simulink model "myFirstRelayModel"  (R2022a)
settings: Solver=VariableStepAuto  StartTime=0.0  StopTime=H  RelTol=1e-3
values from neighbouring files (symbols this model uses):
  Ts = 1    [init.m]    (also in myFirstExtractedData.m; myFirstRelay.m = 0.1; myFirstRelayWithThreeOutputs.m = 0.1)
settings Model: Creator=mrnel  LastModifiedBy=mrnel

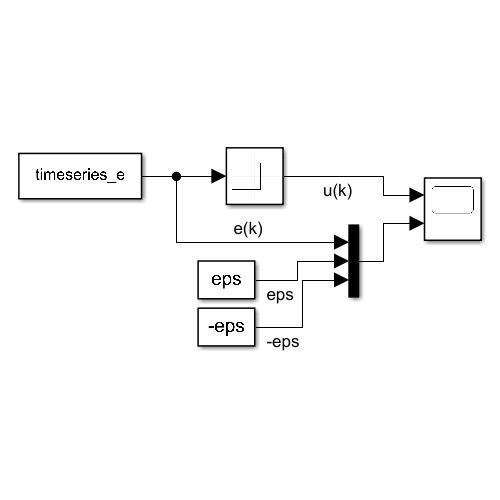
[thumbnail: Simulink's stored preview of the top-level diagram]
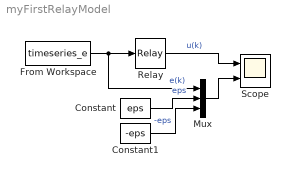
== system myFirstRelayModel ==
  Constant : Constant  Value=eps
  Constant1 : Constant  Value=-eps
  From Workspace : FromWorkspace  VariableName=timeseries_e  SampleTime=Ts
  Mux : Mux  Inputs=3
  Relay : Relay  OffSwitchValue=-eps  OnOutputValue=u_ON  OffOutputValue=u_OFF
  Scope : Scope  NumInputPorts=2
  wires:
  From Workspace/1 -> Mux/1, Relay/1  "e(k)"
  Relay/1 -> Scope/1  "u(k)"
  Constant/1 -> Mux/2  "eps"
  Constant1/1 -> Mux/3  "-eps"
  Mux/1 -> Scope/2
